simulink model "sldemo_househeat"  (R2016b)
settings: Solver=ode45  StartTime=0.0  StopTime=48  FixedStep=1  RelTol=1e-3  AbsTol=1e-6
model workspace (MATLAB code in the model file):
  | % load initial conditions and physical properties from file
  | 
  | sldemo_househeat_data
undefined symbols (not defined in the file or in its folder): c, cost, M, Mdot, Req, THeater, TinIC
libraries: simulink x8, simulink_extras x3
Description:
  | Thermal Model of a House
  | 
  | This demo illustrates how you can use Simulink(R) to create the thermal model of
  | a house. This system models the outdoor environment, the thermal
  | characteristics of the house, and the house heating system.
  | 
  | The sldemo_househeat_data.m file initializes data in the model workspace.
  | To make changes, you can edit the model workspace directly or edit the MATLAB(R) file
  | and re-load the model workspace.
  | 
  | To view the model workspace, select View > Model Explorer
  | from the Simulink editor.
  | 
  | Note: Time is given in units of hours
settings Model: ExtModeTrigMode=oneshot  ExtModeArmWhenConnect=off  ExtModeAutoUpdateStatusClock=off  Creator=The MathWorks, Inc.  LastModifiedBy=GM
settings DataIOCC: ExternalInput=[]  InitialState=[]  SaveFormat=Array  SaveOutput=off  SaveTime=off  SignalLoggingName=sldemo_househeat_output
settings OptimizationCC: BlockReduction=off  BooleanDataType=off  ExpressionDepthLimit=2147483647  InitFltsAndDblsToZero=on  LifeSpan=inf  BufferReusableBoundary=off
settings DebuggingCC: SaveWithParameterizedLinksMsg=none  UnderspecifiedInitializationDetection=Classic  MergeDetectMultiDrivingBlocksExec=none  SignalResolutionControl=TryResolveAllWithWarning  MultiTaskDSMMsg=warning  MultiTaskCondExecSysMsg=none  IntegerOverflowMsg=none  FcnCallInpInsideContextMsg=warning  BusObjectLabelMismatch=none  StateNameClashWarn=warning  SFUnexpectedBacktrackingDiag=warning  SFNoUnconditionalDefaultTransitionDiag=warning  SFExecutionAtInitializationDiag=none  IntegerSaturationMsg=none
settings HardwareCC: ProdBitPerPointer=32  ProdBitPerSizeT=32  ProdBitPerPtrDiffT=32  ProdLargestAtomicFloat=None  ProdIntDivRoundTo=Undefined  ProdEndianess=Unspecified  ProdWordSize=32  ProdHWDeviceType=32-bit Generic  TargetUnknown=on
settings ModelReferenceCC: PropagateSignalLabelsOutOfModel=off
settings GRTTargetCC: TargetFcnLib=ansi_tfl_tmw.mat  TargetLangStandard=C89/C90 (ANSI)  GeneratePreprocessorConditionals=Disable all  CombineOutputUpdateFcns=off  GRTInterface=on
settings ConfigComp: CovMetricSettings=dw  CovHtmlReporting=on  CovSaveCumulativeToWorkspaceVar=on  CovSaveSingleToWorkspaceVar=on  CovExternalEMLEnable=off

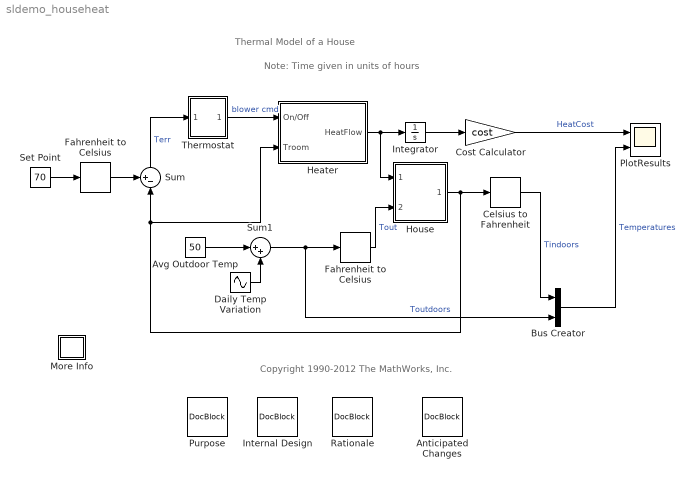
== system sldemo_househeat ==
  note: Thermal Model of a House
  note: Copyright 1990-2012 The MathWorks, Inc.
  note: Note: Time given in units of hours
  Anticipated Changes : simulink/Model-Wide Utilities/DocBlock  Description=This is the Anticipated Changes which should describe alterations that may need to be made to the system.  DocumentType=Text
      content=|
      | This particular model is designed to calculate the heating costs only.
      | If the temperature of the outside air is higher than the room temperature,
      | the room temperature will exceed the desired "Set Point".
      |
      |
      | You can modify this model to include an air conditioner. You can implement the air conditioner as a modified heater.
      | To do this, add parameters like the following to sldemo_househeat_data.m.
      |
      |
      | -Cold air output
      |
      | -Temperature of the stream from the air conditioner
      |
      | -Air conditioner efficiency
      |
      |
      | You would also need to modify the thermostat to control both the air conditioner and the heater.
  Avg Outdoor Temp : Constant  Value=50
  Bus Creator : BusCreator  Inputs=2
  Celsius to Fahrenheit : simulink_extras/Transformations/Celsius to Fahrenheit
  Cost Calculator : Gain  Gain=cost  SaturateOnIntegerOverflow=on  OutDataTypeStr=Inherit: Same as input  ParamDataTypeStr=Inherit: Same as input
  Daily Temp Variation : Sin  Amplitude=15  Frequency=2*pi/24  SampleTime=0
  Fahrenheit to Celsius : simulink_extras/Transformations/Fahrenheit to Celsius
  "Fahrenheit to Celsius " : simulink_extras/Transformations/Fahrenheit to Celsius
  Heater : Subsystem
  House : Subsystem
      mask Display: image(fullfile(matlabroot,'toolbox','simulink','simdemos','simgeneral','images','HouseHeatHousePix.svg'))
  Integrator : Integrator
  Internal Design : simulink/Model-Wide Utilities/DocBlock  Description=This is the Internal Design which should specify how the internal structure of the system fulfills its purpose.  DocumentType=RTF
  More Info : Subsystem
      settings: OpenFcn=showdemo(bdroot(gcb))
      mask Display: disp('?')
  PlotResults : Scope  NumInputPorts=2
  Purpose : simulink/Model-Wide Utilities/DocBlock  Description=This is the Purpose which should specify what the system is designed to accomplish.  DocumentType=Text
      content=|
      | % This is the Purpose which should specify what the system is designed to accomplish.
      | % It should explain the need of the system.
      | %
      | % ---------------Summary of recognized syntax for this text----------------
      | % Lines leading with a "%" will be ignored when the report is generated.
      | %
      | % Creating Links:
      | %   [goto=myLinkID]Clicking this text would move the cursor in the report to the anchor with a LinkID of "myLinkID".[/goto]
      | %   [anchor=myLinkID]The above link would lead to here.[/anchor]
      | %   [url=externalLink]Clicking this text will open an external link, externalLink. (E.g. http://www.mathworks.com/)[/url]
      | %
      | % Adding Images:
      | %   [image=imagePath]imageTitle[/image]
      | %
      | % When you want a new line in the report hit enter twice (a single new line in this document is ignored for readability purposes).
      | %
      | % Any of the lines you see here by default may be removed.
      |
      | The purpose of this system is to model the outdoor environment,
      | the thermal characteristics of the house,
      | and the house heating system.
      | See
      | [url=https://www.mathworks.com/help/simulink/examples/thermal-model-of-a-house.html?s_tid=gn_loc_drop]The MathWorks[/url]
      | page on this model for further details from those provided in this example.
  Rationale : simulink/Model-Wide Utilities/DocBlock  Description=This is the Rationale which should justify why design decisions were made.  DocumentType=Text
      content=|
      | This design was made with separate subsystems
      | for the thermostat, heater, and house
      | in order to increase readability of the model
      | and to modularize the different parts.
  Set Point : Constant  Value=70
  Sum : Sum  Inputs=+-|  SaturateOnIntegerOverflow=on  InputSameDT=on  OutDataTypeStr=Inherit: Same as first input
  Sum1 : Sum  Inputs=|++  SaturateOnIntegerOverflow=on  InputSameDT=on  OutDataTypeStr=Inherit: Same as first input
  Thermostat : Subsystem
      mask Display: image(fullfile(matlabroot,'toolbox','simulink','simdemos','simgeneral','images','HouseHeatThermostatPix.svg'))
  wires:
  Integrator/1 -> Cost Calculator/1
  Thermostat/1(Blower switch) -> Heater/1(On/Off)  "blower cmd"
  Sum/1 -> Thermostat/1(Terr)  "Terr"
  House/1(Room Temp Troom) -> Celsius to Fahrenheit/1, Heater/2(Troom), Sum/2
  Daily Temp Variation/1 -> Sum1/2
  Sum1/1 -> Fahrenheit to Celsius/1, Bus Creator/2  "Toutdoors"
  Avg Outdoor Temp/1 -> Sum1/1
  Celsius to Fahrenheit/1 -> Bus Creator/1  "Tindoors"
  Fahrenheit to Celsius/1 -> House/2(Outdoor Temp Tout)  "Tout"
  Heater/1(HeatFlow) -> Integrator/1, House/1(Heater QDot In)
  Bus Creator/1 -> PlotResults/2  "Temperatures"
  Cost Calculator/1 -> PlotResults/1  "HeatCost"
  "Fahrenheit to Celsius "/1 -> Sum/1
  Set Point/1 -> "Fahrenheit to Celsius "/1

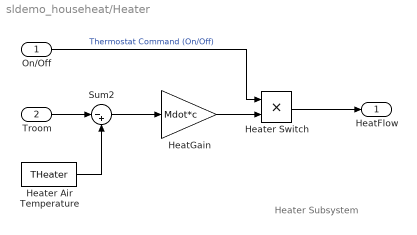
== system sldemo_househeat/Heater ==
  note: Heater Subsystem
  On/Off : Inport
  Troom : Inport  Port=2
  HeatGain : Gain  Gain=Mdot*c
  Heater Air Temperature : Constant  Value=THeater
  Heater Switch : Product  RndMeth=Zero
  Sum2 : Sum  Inputs=|-+
  HeatFlow : Outport
  wires:
  Heater Air Temperature/1 -> Sum2/2
  Troom/1 -> Sum2/1
  Sum2/1 -> HeatGain/1
  On/Off/1 -> Heater Switch/1  "Thermostat Command (On/Off)"
  HeatGain/1 -> Heater Switch/2
  Heater Switch/1 -> HeatFlow/1

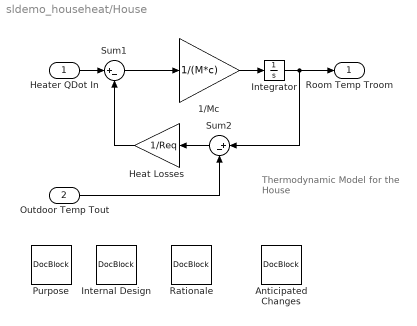
== system sldemo_househeat/House ==
  note: Thermodynamic Model
      | for the House
  Heater QDot In : Inport
  Outdoor Temp Tout : Inport  Port=2
  1/Mc : Gain  Gain=1/(M*c)  SaturateOnIntegerOverflow=on  OutDataTypeStr=Inherit: Same as input  ParamDataTypeStr=Inherit: Same as input
  Anticipated Changes : simulink/Model-Wide Utilities/DocBlock  Description=This is the Anticipated Changes which should describe alterations that may need to be made to the system.  DocumentType=Text
      content=|
      | None.
  Heat Losses : Gain  Gain=1/Req  SaturateOnIntegerOverflow=on  OutDataTypeStr=Inherit: Same as input  ParamDataTypeStr=Inherit: Same as input
  Integrator : Integrator  InitialCondition=TinIC
  Internal Design : simulink/Model-Wide Utilities/DocBlock  Description=This is the Internal Design which should specify how the internal structure of the system fulfills its purpose.  DocumentType=Text
      content=|
      | The environment is modelled as a heat sink with infinite heat capacity and time varying temperature Tout.
      | The constant block "Avg Outdoor Temp" specifies the average air temperature outdoors.
      | The "Daily Temp Variation" Sine Wave block generates daily temperature fluctuations of outdoor temperature.
  Purpose : simulink/Model-Wide Utilities/DocBlock  Description=This is the Purpose which should specify what the system is designed to accomplish.  DocumentType=RTF
  Rationale : simulink/Model-Wide Utilities/DocBlock  Description=This is the Rationale which should justify why design decisions were made.  DocumentType=Text
      content=|
      | A feedback loop is used to model the house
      | since its change in temperature depends on the
      | the previous state.
  Sum1 : Sum  Inputs=|+-  SaturateOnIntegerOverflow=on  InputSameDT=on  OutDataTypeStr=Inherit: Same as first input
  Sum2 : Sum  Inputs=|+-  SaturateOnIntegerOverflow=on  InputSameDT=on  OutDataTypeStr=Inherit: Same as first input
  Room Temp Troom : Outport  InitialOutput=0
  wires:
  Outdoor Temp Tout/1 -> Sum2/2
  Heater QDot In/1 -> Sum1/1
  Sum1/1 -> 1/Mc/1
  Sum2/1 -> Heat Losses/1
  Heat Losses/1 -> Sum1/2
  1/Mc/1 -> Integrator/1
  Integrator/1 -> Sum2/1, Room Temp Troom/1

== system sldemo_househeat/More Info ==

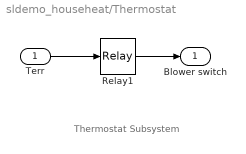
== system sldemo_househeat/Thermostat ==
  note: Thermostat Subsystem
  Terr : Inport
  Relay1 : Relay  OnSwitchValue=5*(5/9)  OffSwitchValue=-5*(5/9)
  Blower switch : Outport  InitialOutput=0
  wires:
  Terr/1 -> Relay1/1
  Relay1/1 -> Blower switch/1
